simulink model "flightControlSystem"  (R2024b)
settings: Solver=ode3  StartTime=0  StopTime=TFinal  FixedStep=Ts  RelTol=1e-3  EnableMultiTasking=on
undefined symbols (not defined in the file): circleCheckNumber, circleHomingGain, circMetricThreshold, codertarget, Controller, DiscIntNeverNeededParam, Discrete, erosionRadius, Estimator, g, gray, init, initialSearchAngle, pixelThreshold, rad, safetyCheckNumber, searchAngle, searchRange, Sensors, strel, takeoffWaitTime, Time, Ts, var_acc_angle_N, var_bias_gyr_N, var_gyro_p_N, Vehicle
libraries: simulink x37, slpidlib x4, ctrlSharedLib x4, sharedtransform x3, dspfdesign x1, visionmorphops x1, parrotlib x1
(part 3 of 3)

== system flightControlSystem/Control System/State Estimator/XY Position Estimator/EstimatorVelocity/xy velocity w//o angular velocity compensation ==
  note: Optical flow raw readings are converted to velocity in m/s based on the estimated altitude
  optical_flow : Inport
  z_estimate : Inport  Port=2
  " " : Product  Inputs=**
  Compare To Constant : simulink/Logic and Bit Operations/Compare To Constant  relop=<  const=200*4  OutDataTypeStr=boolean
  Counter Free-Running : simulink/Sources/Counter Free-Running  NumBits=32  tsamp=-1
  Gain : Gain  Gain=-1
  Select dxy : Selector  InputPortWidth=3  IndexOptions=Index vector (dialog)  Indices=[1 2]  OutputSizes=1
  Switch : Switch  Criteria=u2 > Threshold  SaturateOnIntegerOverflow=off  InputSameDT=off
  opticalFlowErrorCorrect : Gain  Gain=1.15
  optical_flow_dx_dy : Outport
  wires:
  Select dxy/1 -> optical_flow_dx_dy/1  "optical_flow_dx_dy"
  " "/1 -> opticalFlowErrorCorrect/1
  opticalFlowErrorCorrect/1 -> Switch/3
  Gain/1 -> " "/2
  Switch/1 -> Select dxy/1
  Counter Free-Running/1 -> Compare To Constant/1
  Compare To Constant/1 -> Switch/2
  optical_flow/1 -> " "/1, Switch/1
  z_estimate/1 -> Gain/1

== matlab function flightControlSystem/Image Processing System/Circle Detection/Circle Detection Algorithm ==
  data: BW input; detectionFlag output; pixelThreshold input; circMetricThreshold input
function detectionFlag = detectCircle(BW,pixelThreshold,circMetricThreshold)

% Inputs:
% BW: Black and White image
% pixelThreshold: Minimum number of white pixels in the image for the algorithm to activate.
% circMetricThreshold: Threshold to decide if the shape is a circle.

detectionFlag = 0;

if(sum(BW(:)) < pixelThreshold)
    return
end

[row,col] = find(BW);

[~,i_left] = min(col);
[~,i_right] = max(col);

left = [col(i_left),row(i_left)];
right = [col(i_right),row(i_right)];

perimeter = norm(left-right);
area = sum(BW(:));

metric = 4*area/perimeter^2/pi;
if(metric > (2-circMetricThreshold))
    detectionFlag = 0;
    return
end
if(metric > circMetricThreshold)
    detectionFlag = 1;
end
end

== matlab function flightControlSystem/Image Processing System/Landing Point Homing/Landing Point Homing Algorithm ==
  data: BW input; command output
 function command = landHoming(BW)

if(isempty(BW))
    command = [0,0];
    return
end

[row,col] = find(BW);
waypoint = [mean(row),mean(col)];
command = waypoint - [60,80];
command(1) = -command(1);
end

== matlab function flightControlSystem/Image Processing System/Line Search/Line Search Algorithm ==
  data: noPathFlag output; pathAngle input; BW input; pathAngle output; searchRange input; searchAngle input
function [noPathFlag,pathAngle] = findPath(pathAngle,BW,searchRange,searchAngle)

noPathFlag = 1;

for angle = 0:11.25:searchAngle
    u1 = [cosd(pathAngle + angle);sind(pathAngle + angle)];
    u2 = [cosd(pathAngle - angle);sind(pathAngle - angle)];
    R1 = [60;80] + round(searchRange * u1);
    R2 = [60;80] + round(searchRange * u2);
    if(BW(R1(1),R1(2)))
        pathAngle = pathAngle + angle;
        noPathFlag = 0;
        break
    end
    if(BW(R2(1),R2(2)))
        pathAngle = pathAngle - angle;
        noPathFlag = 0;
        break
    end
end

% If a new path angle is not found, pass the old path angle
if(noPathFlag == 1)
    return
end

% Limit path angle to 0-360 degrees
if(pathAngle < 0)
    pathAngle = 360 + pathAngle;
end
if(pathAngle > 360)
    pathAngle = pathAngle - 360;
end

end

== matlab function flightControlSystem/Image Processing System/MATLAB Function4 ==
  data: path_angle input; direction_vector output
function direction_vector = computeDirectionVector(path_angle)
    % Compute the direction vector from the path angle
    direction_vector = [-cos(path_angle) sin(path_angle)];
end

== matlab function flightControlSystem/Image Processing System/MATLAB Function5 ==
  data: detectionFlag input; LandingFlag output; circleCheckNumber input
function LandingFlag = landing_check(detectionFlag, circleCheckNumber)
    persistent counter prevLandingFlag;
    
    if isempty(counter)
        counter = 0;
    end
    if isempty(prevLandingFlag)
        prevLandingFlag = 0;
    end
    
    if detectionFlag
        counter = counter + 1;
    end

    if counter >= circleCheckNumber
        currentLandingFlag = 1;
    else
        currentLandingFlag = 0;
    end

    LandingFlag = prevLandingFlag;
    prevLandingFlag = currentLandingFlag;
end

== matlab function flightControlSystem/Image Processing System/MATLAB Function ==
  data: R input; outR output; G input; B input; outG output; outB output
function [outR, outG, outB]= thresholdRedChannel(R, G, B)
%#codegen
% R, G, B: Ayrı ayrı 2D (rows x cols) uint8 matrisler
% Bu fonksiyon, kırmızı kanalı threshold'un üstünde olan piksellerin
% orijinal R, G, B değerlerini korur, altındakileri siyah yapar.

    % Eşik değeri
    threshold = 150;

    % Görüntü boyutlarını al
    [rows, cols] = size(R);

    % Çıkış resmini (RGB) sıfırlar (uint8 türünde 3D matris)
    out = zeros(rows, cols, 3, 'uint8');

    % Eşik üstü olan pikseller için maske oluştur
    mask = R > threshold;  % mantıksal (logical) matris

    % Mantıksal mask'i uint8'e çevirerek piksel bazında çarpma yapıyoruz:
    % - Maske 1 ise orijinal değeri koru, 0 ise siyah yap.
    mask_uint8 = uint8(mask);

    % Kırmızı kanal
    outR = R .* mask_uint8;
    % Yeşil kanal
    outG = G .* mask_uint8;
    % Mavi kanal
    outB = B .* mask_uint8;
end

== matlab function flightControlSystem/Control System/Controller/Position Controller/Position error transformation (Earth to Body frame) ==
  data: yaw input; xy_err_earth input; xy_err_body output
function xy_err_body = fcn(yaw,xy_err_earth)

transformation = [cos(yaw), sin(yaw); -sin(yaw),  cos(yaw)];
xy_err_body = transformation * xy_err_earth;


end

== matlab function flightControlSystem/Image Processing System/Binarization ==
  data: R input; binaryImage output; G input; B input
function binaryImage = Binarization(R, G, B)
    % RGB kanallarını birleştirerek renkli görüntü oluştur
    rgbImage = cat(3, R, G, B);

    % Kanal eşik değerleri (Histogram analizine göre belirlenmiş)
    redMin = 0;    redMax = 255;
    greenMin = 9;  greenMax = 255;
    blueMin = 0;   blueMax = 255;

    % Belirlenen eşik değerleriyle maske oluştur
    mask = (rgbImage(:,:,1) >= redMin) & (rgbImage(:,:,1) <= redMax) & ...
           (rgbImage(:,:,2) >= greenMin) & (rgbImage(:,:,2) <= greenMax) & ...
           (rgbImage(:,:,3) >= blueMin) & (rgbImage(:,:,3) <= blueMax);

    % Ters çevirerek ikili (binarized) görüntüyü oluştur
    binaryImage = ~mask;
end

== matlab function flightControlSystem/Image Processing System/NoiseFilter ==
  data: BW input; filteredBW output
function filteredBW = NoiseFilter(BW)
    %%%% Gürültü Filtreleme Parametreleri
    % Eşik değeri (Daha düşük değer = Daha fazla filtreleme)
    filterThreshold = 3;

    % Çıktı görüntüsünün boyutları
    imageWidth = 158;
    imageHeight = 118; 

    % Sonuç görüntüsü (sıfırlanmış matris)
    filteredBW = zeros(imageHeight, imageWidth);

    % 3x3 Kutu Filtresi Uygulama
    for row = 2:(imageHeight + 1)
        for col = 2:(imageWidth + 1)
            % 3x3 bölgedeki toplam piksel değerini hesapla
            neighborhoodSum = sum(BW(row-1:row+1, col-1:col+1), 'all');

            % Eşik değerine göre karar ver
            if neighborhoodSum > filterThreshold
                filteredBW(row-1, col-1) = 1;
            else
                filteredBW(row-1, col-1) = 0;
            end
        end
    end
end

== matlab function flightControlSystem/Image Processing System/MATLAB Function1 ==
  data: BW_F input; BW_B_LESS output
function BW_B_LESS = Borderless(BW_F)
    % Kenarlara temas eden nesneleri kaldıran fonksiyon
    
    % === 1️⃣ Parametreleri Tanımla ===
    Border_size = 5;  % Kenardan kaç piksel içeriye kadar kontrol edilecek
    [Height, Width] = size(BW_F);  % Görüntünün boyutlarını al
    
    % Çıktı görüntüsünü başlat
    BW_B_LESS = BW_F;

    % === 2️⃣ Kenarlardaki Pikselleri İşaretle (-1) ===
    BW_F(1:Border_size, :) = -1;  % Üst kenar
    BW_F(end-Border_size+1:end, :) = -1;  % Alt kenar
    BW_F(:, 1:Border_size) = -1;  % Sol kenar
    BW_F(:, end-Border_size+1:end) = -1;  % Sağ kenar

    % === 3️⃣ Kenarlara Temas Eden Nesneleri Bul ve İşaretle (-1) ===
    directions = [-1 0; 1 0; 0 -1; 0 1; -1 -1; -1 1; 1 -1; 1 1]; % 8 yönlü komşular

    for pass = 1:4  % 4 yönden tarama yap
        for i = Border_size+1:Height-Border_size
            for j = Border_size+1:Width-Border_size
                if BW_F(i,j) == 1  % Eğer nesne pikseli ise
                    for d = 1:8  % 8 komşuyu kontrol et
                        ni = i + directions(d,1);
                        nj = j + directions(d,2);
                        if BW_F(ni, nj) == -1
                            BW_F(i,j) = -1;  % Kenara bağlı olduğu için işaretle
                            break;
                        end
                    end
                end
            end
        end
        BW_F = flipud(fliplr(BW_F)); % Görüntüyü çevirerek 4 yönden kontrol et
    end

    % === 4️⃣ İşaretlenmiş Pikselleri (Kenardaki Nesneleri) Sıfırla ===
    BW_B_LESS(BW_F == -1) = 0;

end

== matlab function flightControlSystem/Image Processing System/MATLAB Function2 ==
  data: binaryImage input; isCircleDetected output; filteredImage output
function [isCircleDetected, filteredImage] = Filter_C_Det(binaryImage)
    %%%% Ayar Parametreleri
    filterThreshold = 4;  % Gürültü filtreleme eşiği (Daha düşükse daha fazla filtrelenir)
    minCirclePixels = 300; % Daire tespiti için gereken minimum beyaz piksel sayısı

    % Görüntü boyutları
    [imageHeight, imageWidth] = size(binaryImage);

    % Filtrelenmiş görüntü için boş matris oluştur
    filteredImage = zeros(imageHeight, imageWidth);

    % Gürültü filtreleme işlemi (3x3 komşuluk kontrolü)
    for row = 2:imageHeight-1
        for col = 2:imageWidth-1
            % 3x3 komşu piksellerin toplamını al
            neighborhoodSum = sum(binaryImage(row-1:row+1, col-1:col+1), 'all');
            
            % Eşik değerden büyükse beyaz (1), değilse siyah (0) yap
            if neighborhoodSum > filterThreshold
                filteredImage(row, col) = 1;
            else
                filteredImage(row, col) = 0;
            end
        end
    end

    % Toplam beyaz piksel sayısına göre daire olup olmadığını kontrol et
    if sum(filteredImage, 'all') > minCirclePixels
        isCircleDetected = 1;  % Daire tespit edildi
    else
        isCircleDetected = 0;  % Daire tespit edilmedi
    end
end

== matlab function flightControlSystem/Image Processing System/MATLAB Function3 ==
  data: BW input; x_incr output; xp input; yp input; y_incr output; Start_End_Flag output
function [x_incr, y_incr, Start_End_Flag] = Radar(BW, xp, yp)
    % Parametreler
    box = 9;  % Tarama penceresi boyutu
    Thrs = box * box / 2;  % Beyaz piksel eşiği
    Red_Srch = 1;  % Tarama çözünürlüğü (derece cinsinden)
    Width = 158;
    Height = 118;
    
    % Görüntünün belirli bir bölgesini işle (kenarları kırp)
    BW2 = BW(:, 20:139);
    
    % Başlangıç değerleri
    Start_End_Flag = 0;
    x_incr = 0;
    y_incr = 0;
    
    % 360 derece boyunca tarama yap
    Angle_detection = zeros(1, 360);
    for i = 0:Red_Srch:359
        % Taramada kullanılan koordinatları hesapla
        x_b_pos = round(xp + cosd(i) * box);
        y_b_pos = round(yp + sind(i) * box);
        
        % Koordinatlar görüntü sınırları içinde mi kontrol et
        if (x_b_pos - (box-1)/2) >= 1 && (y_b_pos - (box-1)/2) >= 1 && ...
           (x_b_pos + (box-1)/2) <= Width && (y_b_pos + (box-1)/2) <= Height
            
            % Kare pencere içinde beyaz pikselleri say
            region = BW2(x_b_pos-((box-1)/2):x_b_pos+((box-1)/2), ...
                         y_b_pos-((box-1)/2):y_b_pos+((box-1)/2));
            white_pixel_count = sum(region(:));
            
            % Eşik değerini geçen alanları belirle
            Angle_detection(i+1) = white_pixel_count >= Thrs;
        end
    end
    
    % Beyaz bölgelerin merkez koordinatlarını belirle
    detected_angles = find(Angle_detection);
    num_detected = length(detected_angles);
    
    % Eğer en az bir nesne algılandıysa, koordinatları hesapla
    if num_detected > 0
        x_centers = xp + cosd(detected_angles) * box;
        y_centers = yp + sind(detected_angles) * box;
        
        % En yakın merkezi belirle
        distances = sqrt((x_centers - xp).^2 + (y_centers - yp).^2);
        [~, min_index] = min(distances);
        
        % Yeni artış değerlerini belirle
        x_incr = x_centers(min_index);
        y_incr = y_centers(min_index);
        Start_End_Flag = 1;
    end
end

== matlab function flightControlSystem/Image Processing System/rgb_to_bw ==
  data: R input; BW output; G input; B input
function BW = RGBtoBW(R,G,B)
    % Giriş resmi I RGB formatında olmalı.
    % R_min, R_max, G_min, G_max, B_min, B_max renk sınırlarıdır.

    % RGB kanallarını ayır
    
    % Her bir renk kanalı için sınırlar içinde olup olmadığını kontrol et
    R_bw = (R >= 127) & (R <= 255);
    G_bw = (G >= 0) & (G <= 151);
    B_bw = (B >= 0) & (B <= 149);

    % Tüm koşullar sağlandığında pikseli beyaz yap, değilse siyah
    BW = R_bw & G_bw & B_bw;

    % BW resmini döndür
end

== stateflow chart flightControlSystem/Control System/Path Planning/Chart ==
  state Land
    during:
    xout = double(xestim)+ double(xRef);
    yout = double(yestim) + double(yRef);
    zout = 0.0;
  state Takeoff
    entry:
    xout = 0;
    yout = 0;
    zout = -1.1;
  state Go
    xout = double(xestim)+ double(xRef);
    yout = double(yestim) + double(yRef);
    zout = -1.1;
  (default) -> Takeoff
  Takeoff -> Go : [after(3,sec)]
  Go -> Land : [landingFlag==1 && sqrt(dx^2 +dy^2+dz^2) <= 0.01 ]
  data: xestim input; yestim input; xRef input; yRef input; landingFlag input; xout output; yout output; zout output; dz input; dx input; dy input
